simulink model "MagLev_NonLinearSys_ResponseToDifferentInputWaveforms"  (R2019b)
settings: Solver=VariableStepAuto  StartTime=0.0  StopTime=40  RelTol=1e-3
libraries: cstblocks x1, simulink x1
settings Model: Creator=Santoshi Kulkarni  LastModifiedBy=Santoshi Kulkarni

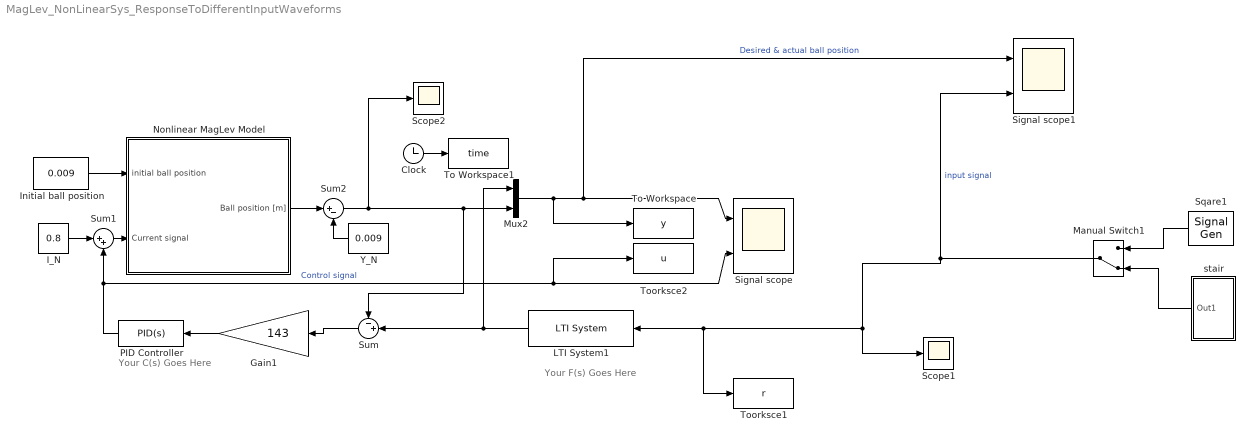
== system MagLev_NonLinearSys_ResponseToDifferentInputWaveforms ==
  note: Your F(s) Goes Here
  note: Your C(s) Goes Here
  Clock : Clock
  Gain1 : Gain  Gain=143
  I_N : Constant  Value=0.8
  Initial ball position : Constant  Value=0.009
  LTI System1 : cstblocks/LTI System  sys=tf(5,[1 5])  IC=[]
  Manual Switch1 : ManualSwitch  CurrentSetting=0
  Mux2 : Mux  Inputs=2
  Nonlinear MagLev Model : Subsystem
  PID Controller : simulink/Continuous/PID Controller  Controller=PID  Form=Parallel  TimeDomain=Continuous-time  SampleTime=-1  IntegratorMethod=Forward Euler  FilterMethod=Forward Euler  ControllerParametersSource=internal  P=-4.45  I=-3.09  D=-0.0532  UseFilter=on  N=1000  TunerSelectOption=Transfer Function Based (PID Tuner App)  InitialConditionSource=internal  InitialConditionForIntegrator=0  InitialConditionForFilter=0  DifferentiatorICPrevScaledInput=0  ExternalReset=none  TrackingMode=off  Kt=1  LimitOutput=off  UpperSaturationLimit=inf  LowerSaturationLimit=-inf  LinearizeAsGain=on  AntiWindupMode=none  Kb=1  POutMin=[]  POutMax=[]  IOutMin=[]  IOutMax=[]  DOutMin=[]  DOutMax=[]  NOutMin=[]  NOutMax=[]  SumOutMin=[]  SumOutMax=[]  SaturationOutMin=[]  SaturationOutMax=[]  PParamMin=[]  PParamMax=[]  IParamMin=[]  IParamMax=[]  DParamMin=[]  DParamMax=[]  NParamMin=[]  NParamMax=[]  KbParamMin=[]  KbParamMax=[]  KtParamMin=[]  KtParamMax=[]  KbOutMin=[]  KbOutMax=[]  KtOutMin=[]  KtOutMax=[]  IntegratorOutMin=[]  IntegratorOutMax=[]  FilterOutMin=[]  FilterOutMax=[]  SumI1OutMin=[]  SumI1OutMax=[]  SumI2OutMin=[]  SumI2OutMax=[]  SumI3OutMin=[]  SumI3OutMax=[]  SumI4OutMin=[]  SumI4OutMax=[]  SumDOutMin=[]  SumDOutMax=[]  DifferentiatorOutMin=[]  DifferentiatorOutMax=[]  FilterDiffOutCoefMin=[]  FilterDiffOutCoefMax=[]  ReciprocalOutMin=[]  ReciprocalOutMax=[]  SumDenOutMin=[]  SumDenOutMax=[]  SumNumOutMin=[]  SumNumOutMax=[]  DivideOutMin=[]  DivideOutMax=[]  IntegratorContinuousStateAttributes=''  IntegratorStateMustResolveToSignalObject=off  IntegratorRTWStateStorageClass=Auto  FilterContinuousStateAttributes=''  FilterStateMustResolveToSignalObject=off  FilterRTWStateStorageClass=Auto  ParallelPVariant=InternalParameters  IdealPVariant=Disabled  IVariant=InternalParameters  DVariant=InternalParameters  IntegratorVariant=Continuous  SatVariant=Disabled  AWVariant=Passthrough  PCopyVariant=Disabled  TRVariant=Disabled  FdbkBlocksVariant=Forward  IdealPFdbkVariant=Disabled  SatFdbkVariant=Disabled  DerivativeFilterVariant=ContFilter  NVariant=InternalParameters  NCopyVariant=Disabled  FilterICVariant=InternalICsFilter  IntegratorICVariant=InternalICs  ExternalResetVariant=Disabled  TRSumVariant=Passthrough  SumFdbkVariant=Disabled  SumVariant=Sum_PID
  Scope1 : Scope
  Scope2 : Scope
  Signal scope : Scope  NumInputPorts=2
  Signal scope1 : Scope  NumInputPorts=2
  Sqare1 : SignalGenerator  WaveForm=square  Amplitude=0.005  Frequency=1/8
  Sum : Sum  Inputs=-+|
  Sum1 : Sum  Inputs=|++
  Sum2 : Sum  Inputs=|+-
  To Workspace : ToWorkspace  VariableName=y  SampleTime=0.01
  To Workspace1 : ToWorkspace  VariableName=time  SampleTime=0.01
  Toorksce1 : ToWorkspace  VariableName=r  SampleTime=0.01
  Toorksce2 : ToWorkspace  VariableName=u  SampleTime=0.01
  Y_N : Constant  Value=0.009
  stair : Subsystem
  wires:
  Sqare1/1 -> Manual Switch1/1
  Clock/1 -> To Workspace1/1
  stair/1(Out1) -> Manual Switch1/2
  Sum2/1 -> Scope2/1, Mux2/2, Sum/1
  Mux2/1 -> Signal scope1/1, Signal scope/1, To Workspace/1  "Desired & actual ball position"
  Sum/1 -> Gain1/1
  Gain1/1 -> PID Controller/1
  LTI System1/1 -> Mux2/1, Sum/2
  Y_N/1 -> Sum2/2
  Manual Switch1/1 -> LTI System1/1, Toorksce1/1, Scope1/1, Signal scope1/2  "input signal"
  Sum1/1 -> Nonlinear MagLev Model/2(Current signal)
  I_N/1 -> Sum1/1
  Nonlinear MagLev Model/1(Ball position [m]) -> Sum2/1
  PID Controller/1 -> Signal scope/2, Toorksce2/1, Sum1/2  "Control signal"
  Initial ball position/1 -> Nonlinear MagLev Model/1(initial ball position)

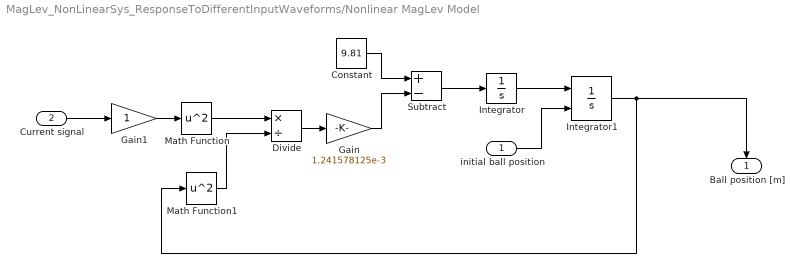
== system MagLev_NonLinearSys_ResponseToDifferentInputWaveforms/Nonlinear MagLev Model ==
  initial ball position : Inport
  Current signal : Inport  Port=2
  Constant : Constant  Value=9.81
  Divide : Product  Inputs=*/
  Gain : Gain  Gain=1.241578125e-3
  Gain1 : Gain
  Integrator : Integrator
  Integrator1 : Integrator  InitialConditionSource=external
  Math Function : Math  Operator=square  SaturateOnIntegerOverflow=on
  Math Function1 : Math  Operator=square  SaturateOnIntegerOverflow=on
  Subtract : Sum  Inputs=+-
  Ball position [m] : Outport
  wires:
  Gain1/1 -> Math Function/1
  Current signal/1 -> Gain1/1
  initial ball position/1 -> Integrator1/2
  Integrator1/1 -> Math Function1/1, Ball position [m]/1
  Integrator/1 -> Integrator1/1
  Subtract/1 -> Integrator/1
  Gain/1 -> Subtract/2
  Divide/1 -> Gain/1
  Math Function1/1 -> Divide/2
  Math Function/1 -> Divide/1
  Constant/1 -> Subtract/1

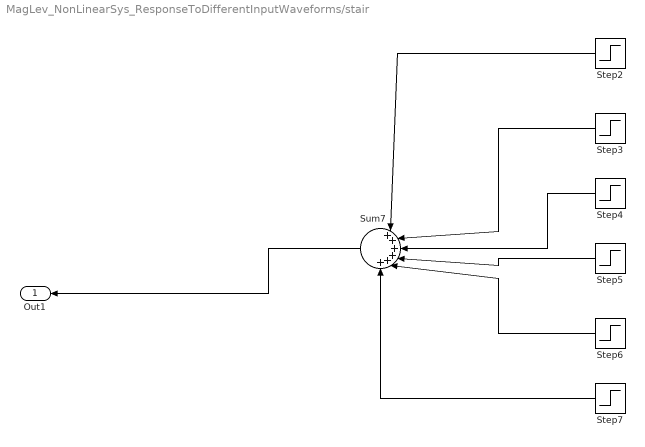
== system MagLev_NonLinearSys_ResponseToDifferentInputWaveforms/stair ==
  Step2 : Step  Time=7  After=0.005  SampleTime=0
  Step3 : Step  Time=14  After=0.005  SampleTime=0
  Step4 : Step  Time=21  After=0.005  SampleTime=0
  Step5 : Step  Time=28  After=0.005  SampleTime=0
  Step6 : Step  Time=35  After=0.005  SampleTime=0
  Step7 : Step  Time=42  After=0.005  SampleTime=0
  Sum7 : Sum  Inputs=|++++++
  Out1 : Outport
  wires:
  Step6/1 -> Sum7/5
  Step3/1 -> Sum7/2
  Step7/1 -> Sum7/6
  Sum7/1 -> Out1/1
  Step5/1 -> Sum7/4
  Step4/1 -> Sum7/3
  Step2/1 -> Sum7/1
